simulink model "blance_leg"  (R2023a)
settings: Solver=VariableStepAuto  StartTime=0.0  StopTime=5  MaxStep=0.24  RelTol=1e-3
undefined symbols (not defined in the file): a11, a12, a13, a14, a15, a16, a21, a22, a23, a24, a25, a26, X, Y, Z
libraries: sm_lib x114, nesl_utility x23, matrix_library x4, slpidlib x2
(part 4 of 4)

== matlab function blance_leg/Subsystem1/MATLAB Function12 ==
  data: k output; a input; length input
function k = get_K(a,length)
   k = polyval(a,length);  
end

== matlab function blance_leg/Subsystem1/MATLAB Function2 ==
  data: k output; a input; length input
function k = get_K(a,length)
   k = polyval(a,length);  
end

== matlab function blance_leg/Subsystem1/MATLAB Function3 ==
  data: k output; a input; length input
function k = get_K(a,length)
   k = polyval(a,length);  
end

== matlab function blance_leg/Subsystem1/MATLAB Function4 ==
  data: k output; a input; length input
function k = get_K(a,length)
   k = polyval(a,length);  
end

== matlab function blance_leg/Subsystem1/MATLAB Function5 ==
  data: k output; a input; length input
function k = get_K(a,length)
   k = polyval(a,length);  
end

== matlab function blance_leg/calc/MATLAB Function1 ==
  data: k output; a input; length input
function k = get_K(a,length)
   k = polyval(a,length);  
end

== matlab function blance_leg/Subsystem1/MATLAB Function6 ==
  data: k output; a input; length input
function k = get_K(a,length)
   k = polyval(a,length);  
end

== matlab function blance_leg/Subsystem1/MATLAB Function7 ==
  data: k output; a input; length input
function k = get_K(a,length)
   k = polyval(a,length);  
end

== matlab function blance_leg/Subsystem1/MATLAB Function8 ==
  data: k output; a input; length input
function k = get_K(a,length)
   k = polyval(a,length);  
end

== matlab function blance_leg/Subsystem1/MATLAB Function9 ==
  data: k output; a input; length input
function k = get_K(a,length)
   k = polyval(a,length);  
end

== matlab function blance_leg/Right Controller/MATLAB Function3 ==
  data: d_phi0 output; J input; d_phi1 input; d_phi2 input; d_L0 output
function [d_phi0,d_L0] = D_PHI0(J,d_phi1,d_phi2)
    q_dot = J*[d_phi1;d_phi2];
    d_L0 = q_dot(1);
    d_phi0 = q_dot(2);
    
end

== matlab function blance_leg/MATLAB Function2 ==
  data: phi2_3 output; L0 input
function phi2_3 = PHI2_3(L0)
    l1=0.15;
    l2=0.25;

    phi2_3 = pi - acos((l1*l1+l2*l2-L0*L0)/(2*l1*l2));
end

== matlab function blance_leg/Left Controller/MATLAB Function4 ==
  data: L0 output; phi1 input; phi2 input; phi0 output
function [L0,phi0] = L0_PHI0(phi1,phi2)
    l1=0.15;
    l2=0.25;

    x_C = l1*cos(phi1) + l2*cos(phi2);
    y_C = l1*sin(phi1) + l2*sin(phi2);
    
    L0 = sqrt(x_C*x_C + y_C*y_C);
    phi0 = atan2(y_C,x_C);
end

== matlab function blance_leg/calc/MATLAB Function2 ==
  data: k output; a input; length input
function k = get_K(a,length)
   k = polyval(a,length);  
end

== matlab function blance_leg/calc/MATLAB Function3 ==
  data: k output; a input; length input
function k = get_K(a,length)
   k = polyval(a,length);  
end

== matlab function blance_leg/calc/MATLAB Function4 ==
  data: k output; a input; length input
function k = get_K(a,length)
   k = polyval(a,length);  
end

== matlab function blance_leg/calc/MATLAB Function5 ==
  data: k output; a input; length input
function k = get_K(a,length)
   k = polyval(a,length);  
end

== matlab function blance_leg/Right Controller/MATLAB Function4 ==
  data: L0 output; phi1 input; phi2 input; phi0 output
function [L0,phi0] = L0_PHI0(phi1,phi2)
    l1=0.15;
    l2=0.25;

    x_C = l1*cos(phi1) + l2*cos(phi2);
    y_C = l1*sin(phi1) + l2*sin(phi2);
    
    L0 = sqrt(x_C*x_C + y_C*y_C);
    phi0 = atan2(y_C,x_C);
end

== matlab function blance_leg/MATLAB Function1 ==
  data: L0 output; phi1 input; phi2 input; phi0 output
function [L0,phi0] = L0_PHI0(phi1,phi2)
    l1=0.15;
    l2=0.25;

    x_C = l1*cos(phi1) + l2*cos(phi2);
    y_C = l1*sin(phi1) + l2*sin(phi2);
    
    L0 = sqrt(x_C*x_C + y_C*y_C);
    phi0 = atan2(y_C,x_C);
end

== matlab function blance_leg/phi format ==
  data: Phi1 output; phi1 input; phi2 input; Phi2 output
function [Phi1,Phi2] = PhiFormat(phi1,phi2)
    Phi1 = -(phi1-pi/2);
    Phi2 = Phi1-phi2;

    Phi1 = pi - Phi1;
    Phi2 = pi - Phi2;
end

== matlab function blance_leg/phi format1 ==
  data: Phi1 output; phi1 input; phi2 input; Phi2 output
function [Phi1,Phi2] = PhiFormat(phi1,phi2)
    Phi1 = -(phi1-pi/2);
    Phi2 = Phi1-phi2;

    Phi1 = pi - Phi1;
    Phi2 = pi - Phi2;
end

== matlab function blance_leg/MATLAB Function4 ==
  data: L0 output; phi1 input; phi2 input; phi0 output
function [L0,phi0] = L0_PHI0(phi1,phi2)
    l1=0.15;
    l2=0.25;

    x_C = l1*cos(phi1) + l2*cos(phi2);
    y_C = l1*sin(phi1) + l2*sin(phi2);
    
    L0 = sqrt(x_C*x_C + y_C*y_C);
    phi0 = atan2(y_C,x_C);
end
